simulink model "metoda2_bezposrednia"  (R2017b)
settings: Solver=VariableStepAuto  StartTime=0.0  StopTime=10  RelTol=1e-3
values from neighbouring files (symbols this model uses):
  A2 = [3.22791678547  1  0; -1.44925930399  0  1; 0.17377394345  0  0]    [matlab.mat]
  B2 = [0.260707487539 -0.289205764977 0.0761198486843]    [matlab.mat]
  Tp = 0.25    [matlab.mat]
  x_start = [3 -2 1]    [matlab.mat]
settings Model: Creator=gulin  LastModifiedBy=gulin

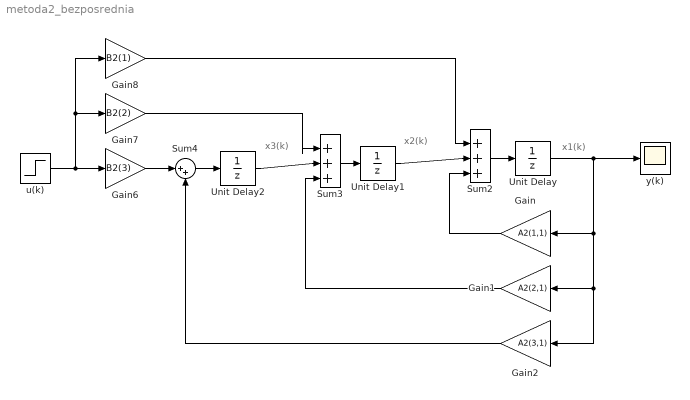
== system metoda2_bezposrednia ==
  note: x1(k)
  note: x3(k)
  note: x2(k)
  Gain : Gain  Gain=A2(1,1)
  Gain1 : Gain  Gain=A2(2,1)
  Gain2 : Gain  Gain=A2(3,1)
  Gain6 : Gain  Gain=B2(3)
  Gain7 : Gain  Gain=B2(2)
  Gain8 : Gain  Gain=B2(1)
  Sum2 : Sum  Inputs=|+++
  Sum3 : Sum  Inputs=|+++
  Sum4 : Sum  Inputs=|++
  Unit Delay : UnitDelay  InitialCondition=x_start(1)  SampleTime=Tp
  Unit Delay1 : UnitDelay  InitialCondition=x_start(2)  SampleTime=Tp
  Unit Delay2 : UnitDelay  InitialCondition=x_start(3)  SampleTime=Tp
  u(k) : Step  SampleTime=0
  y(k) : Scope
  wires:
  Unit Delay/1 -> y(k)/1, Gain2/1, Gain1/1, Gain/1
  Sum2/1 -> Unit Delay/1
  Sum3/1 -> Unit Delay1/1
  Sum4/1 -> Unit Delay2/1
  Gain2/1 -> Sum4/2
  Gain6/1 -> Sum4/1
  u(k)/1 -> Gain8/1, Gain7/1, Gain6/1
  Unit Delay2/1 -> Sum3/2
  Gain7/1 -> Sum3/1
  Gain1/1 -> Sum3/3
  Gain8/1 -> Sum2/1
  Gain/1 -> Sum2/3
  Unit Delay1/1 -> Sum2/2
